simulink model "DVA"  (R2020b)
settings: Solver=VariableStepAuto  StartTime=0.0  StopTime=50.0  RelTol=1e-3
undefined symbols (not defined in the file): b, K1, k12, M1, M2
settings Model: Creator=Shubham  LastModifiedBy=Shubham
settings DataIOCC: OutputSaveName=output

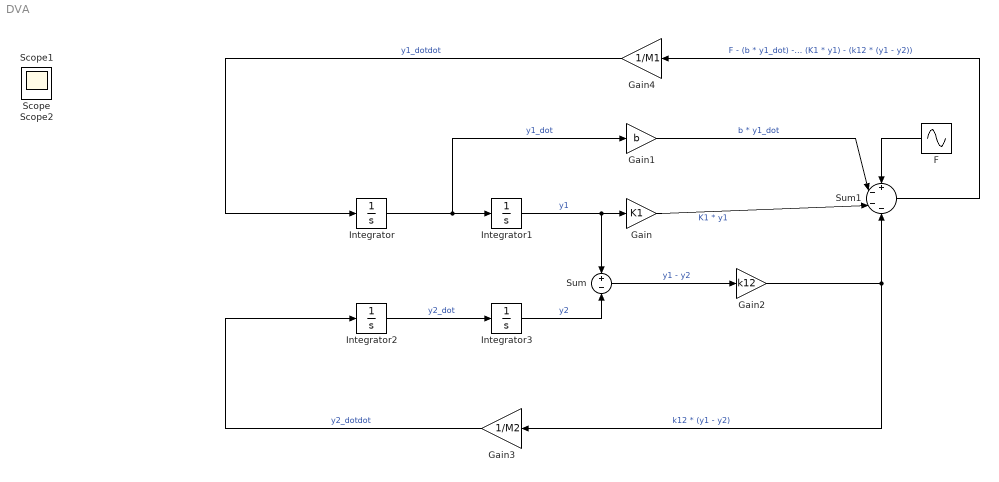
== system DVA ==
  F : Sin  Amplitude=2  Frequency=10  SampleTime=0
  Gain : Gain  Gain=K1
  Gain1 : Gain  Gain=b
  Gain2 : Gain  Gain=k12
  Gain3 : Gain  Gain=1/M2
  Gain4 : Gain  Gain=1/M1
  Integrator{,1..3} (4 alike) : Integrator
  Sum : Sum  Inputs=+-
  Sum1 : Sum  Inputs=+---
  Scope : Scope
  Scope1 : Scope
  Scope2 : Scope
  wires:
  Integrator/1 -> Gain1/1, Integrator1/1  "y1_dot"
  Gain4/1 -> Integrator/1  "y1_dotdot"
  Integrator1/1 -> Gain/1, Sum/1  "y1"
  Gain/1 -> Sum1/3  "K1 * y1"
  Gain1/1 -> Sum1/2  "b * y1_dot"
  Integrator2/1 -> Integrator3/1  "y2_dot"
  Gain3/1 -> Integrator2/1  "y2_dotdot"
  Integrator3/1 -> Sum/2  "y2"
  Sum/1 -> Gain2/1  "y1 - y2"
  Gain2/1 -> Sum1/4, Gain3/1  "k12 * (y1 - y2)"
  Sum1/1 -> Gain4/1  "F - (b * y1_dot) - (K1 * y1) - (k12 * (y1 - y2))"
  F/1 -> Sum1/1
